simulink model "chap5_4sim"  (Simulink 7.7)
settings: Solver=ode45  StartTime=0.0  StopTime=20  FixedStep=0.001  RelTol=1e-3
settings Model: Creator=hp  LastModifiedBy=ljk  ExtModeTrigMode=oneshot  ExtModeArmWhenConnect=off
settings DataIOCC: LimitDataPoints=off  SignalLoggingName=sigsOut
settings OptimizationCC: BooleanDataType=off  InitFltsAndDblsToZero=on
settings DebuggingCC: SaveWithParameterizedLinksMsg=none  SignalResolutionControl=TryResolveAllWithWarning  SolverPrmCheckMsg=none  MultiTaskDSMMsg=warning  MultiTaskCondExecSysMsg=none  StrictBusMsg=None
settings HardwareCC: TargetUnknown=on
settings RTWCC: IncludeERTFirstTime=on
settings GRTTargetCC: TargetFcnLib=ansi_tfl_tmw.mat

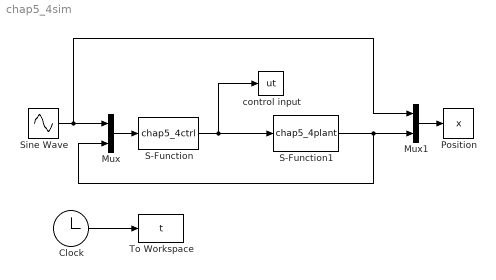
== system chap5_4sim ==
  Clock : Clock
      settings: Decimation=10
  Mux : Mux  Inputs=2
  Mux1 : Mux  Inputs=2
  Position : ToWorkspace  VariableName=x  SampleTime=-1  SaveFormat=Array
  S-Function : S-Function  FunctionName=chap5_4ctrl  EnableBusSupport=off
  S-Function1 : S-Function  FunctionName=chap5_4plant  EnableBusSupport=off
  Sine Wave : Sin  SampleTime=0
  To Workspace : ToWorkspace  VariableName=t  SampleTime=-1  SaveFormat=Array
  control input : ToWorkspace  VariableName=ut  SampleTime=-1  SaveFormat=Array
  wires:
  S-Function/1 -> S-Function1/1, control input/1
  S-Function1/1 -> Mux/2, Mux1/2
  Clock/1 -> To Workspace/1
  Mux/1 -> S-Function/1
  Sine Wave/1 -> Mux/1, Mux1/1
  Mux1/1 -> Position/1
